simulink model "audio"  (Simulink 6.6)
settings: Solver=VariableStepDiscrete  StartTime=0.0  StopTime=15  RelTol=1e-3
PreLoadFcn:
  | Tsysclk=1/24000000;
  | Fs = 48000;
  | code_a = [0 0 0 0 1];
  | code_b = [0 0 0 1 0];
  | code_c = [0 0 0 1 1];
  | code_d = [1 0 1 1 1];
  | sum_filter_taps = ones(1,31);
libraries: xbsIndex_r4 x57, dspwin32 x2, simulink x1
settings Model: Creator=lcrockett  LastModifiedBy=lcrockett
settings OptimizationCC: InlineParams=on  InlineInvariantSignals=on
settings DebuggingCC: SignalResolutionControl=TryResolveAllWithWarning  MultiTaskDSMMsg=warning  MultiTaskCondExecSysMsg=none  StrictBusMsg=None
settings HardwareCC: TargetHWDeviceType=32-bit Generic  ProdEqTarget=off
settings RTWCC: IncludeERTFirstTime=on

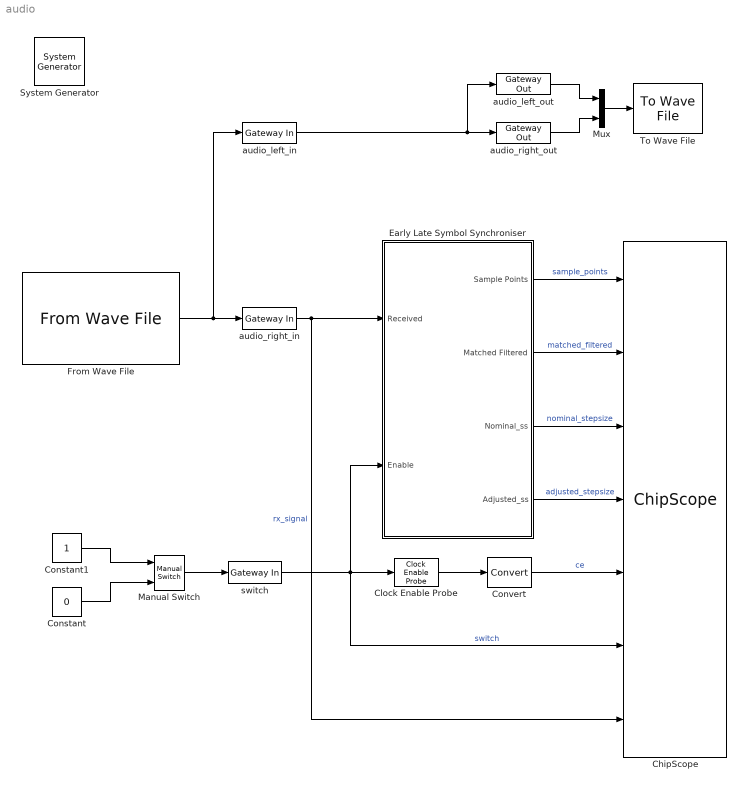
== system audio ==
  " System Generator" : xbsIndex_r4/ System Generator  Tag=genX  SystemSampleTime=-1  xilinxfamily=virtex2p  part=xc2vp30  speed=-7  package=ff896  synthesis_tool=XST  clock_wrapper=Clock Enables  directory=./audio_earlylate  testbench=off  simulink_period=Tsysclk  sysclk_period=50  dcm_input_clock_period=100  incr_netlist=off  trim_vbits=Everywhere in SubSystem  dbl_ovrd=According to Block Masks  core_generation=According to Block Masks  run_coregen=off  deprecated_control=off  eval_field=0  block_type=sysgen
      settings: block_version=8.2
  ChipScope : xbsIndex_r4/ChipScope  num_trig_ports=7  current_port=5  show_trig_port=0  match_units=1  match_type=Extended  data_is_trigger=on  num_data_ports=4  data_depth=16384  SRL16s=on  match_type_t0=1  match_type_t1=3  match_type_t2=3  match_type_t3=3  match_type_t4=3  match_type_t5=3  match_type_t6=3  match_type_t7=1  match_type_t8=1  match_type_t9=1  match_type_t10=1  match_type_t11=1  match_type_t12=1  match_type_t13=1  match_type_t14=1  match_type_t15=1  match_units_t0=1  match_units_t1=1  match_units_t2=1  match_units_t3=1  match_units_t4=1  match_units_t5=1  match_units_t6=1  match_units_t7=1  match_units_t8=1  match_units_t9=1  match_units_t10=1  match_units_t11=1  match_units_t12=1  match_units_t13=1  match_units_t14=1  match_units_t15=1  dbl_ovrd=0  block_type=chipscope
      settings: infoedit="Enables run-time debugging and verification of signals by inserting ChipScope Pro ICON and ILA cores.<br><br>  Restrictions: <br>Only one ChipScope core can be instantiated in a System Generator design.This block cannot be used at the same time as JTAG hardware co-simulation.A design or subsystem containing a ChipScope block must have at least one output port."  block_version=10.1.2
  Clock Enable Probe : xbsIndex_r4/Clock Enable Probe  block_type=ceprobe
      settings: infoedit="Clock enable extractor.  Produces a Boolean output that mirrors the hardware clock enable associated with the input sample rate.<P><P>Hardware notes: in hardware this block costs nothing."  block_version=10.1.2
  Constant : Constant  Value=0  SampleTime=Tsysclk*500
  Constant1 : Constant  SampleTime=Tsysclk*500
  Convert : xbsIndex_r4/Convert  arith_type=Unsigned  n_bits=1  bin_pt=0  quantization=Truncate  overflow=Wrap  latency=0  dbl_ovrd=off  pipeline=off  block_type=convert
      settings: block_version=10.1.2
  Early Late Symbol Synchroniser : Subsystem
  From Wave File : dspwin32/From Wave File  FileName=baseband_audio  SamplesPerFrame=1  MinBufSize=128  dType=double  bLoop=off  timesToPlay=1  restartMode=immediately after last sample  firstSampleOutput=off  lastSampleOutput=off
  Manual Switch : simulink/Signal Routing/Manual Switch  SystemSampleTime=-1  sw=0  action=0  varsize=off
  Mux : Mux  Inputs=2
  To Wave File : dspwin32/To Wave File  filename=audio  sampleWidth=16  MinNumSamples=256
  audio_left_in : xbsIndex_r4/Gateway In  arith_type="Signed  (2's comp)"  n_bits=16  bin_pt=14  quantization="Round  (unbiased: +/- Inf)"  overflow=Saturate  period=Tsysclk*500  dbl_ovrd=off  timing_constraint=None  locs_specified=off  LOCs={}  block_type=gatewayin
      settings: infoedit="Gateway in block.  Converts inputs of type Simulink integer, double and fixed point to  Xilinx fixed point type.<P><P>Hardware notes:  In hardware these blocks become top level input ports."  xl_area=[0 0 0 0 16 0 0]  block_version=VER_STRING_GOES_HERE
  audio_left_out : xbsIndex_r4/Gateway Out  hdl_port=on  timing_constraint=None  locs_specified=off  LOCs={}  block_type=gatewayout
      settings: infoedit="Gateway out block.  Converts Xilinx fixed point inputs into ouputs of type Simulink integer, double, or fixed point.<P><P>Hardware notes:  In hardware these blocks become top level output ports or are discarded, depending on how they are configured."  xl_area=[0 0 0 0 16 0 0]  block_version=VER_STRING_GOES_HERE
  audio_right_in : xbsIndex_r4/Gateway In  arith_type="Signed  (2's comp)"  n_bits=16  bin_pt=14  quantization="Round  (unbiased: +/- Inf)"  overflow=Saturate  period=Tsysclk*500  dbl_ovrd=off  timing_constraint=None  locs_specified=off  LOCs={}  block_type=gatewayin
      settings: infoedit="Gateway in block.  Converts inputs of type Simulink integer, double and fixed point to  Xilinx fixed point type.<P><P>Hardware notes:  In hardware these blocks become top level input ports."  xl_area=[0 0 0 0 16 0 0]  block_version=VER_STRING_GOES_HERE
  audio_right_out : xbsIndex_r4/Gateway Out  hdl_port=on  timing_constraint=None  locs_specified=off  LOCs={}  block_type=gatewayout
      settings: infoedit="Gateway out block.  Converts Xilinx fixed point inputs into ouputs of type Simulink integer, double, or fixed point.<P><P>Hardware notes:  In hardware these blocks become top level output ports or are discarded, depending on how they are configured."  xl_area=[0 0 0 0 16 0 0]  block_version=VER_STRING_GOES_HERE
  switch : xbsIndex_r4/Gateway In  arith_type=Boolean  n_bits=16  bin_pt=14  quantization="Round  (unbiased: +/- Inf)"  overflow=Saturate  period=Tsysclk*500  dbl_ovrd=off  timing_constraint=None  locs_specified=off  LOCs={}  block_type=gatewayin
      settings: infoedit="Gateway in block.  Converts inputs of type Simulink integer, double and fixed point to  Xilinx fixed point type.<P><P>Hardware notes:  In hardware these blocks become top level input ports."  xl_area=[0 0 0 0 16 0 0]  block_version=VER_STRING_GOES_HERE
  wires:
  From Wave File/1 -> audio_left_in/1, audio_right_in/1
  audio_right_out/1 -> Mux/2
  audio_left_out/1 -> Mux/1
  Mux/1 -> To Wave File/1
  switch/1 -> Clock Enable Probe/1, Early Late Symbol Synchroniser/2(Enable), ChipScope/6  "switch"
  Manual Switch/1 -> switch/1
  Constant1/1 -> Manual Switch/1
  Constant/1 -> Manual Switch/2
  audio_left_in/1 -> audio_left_out/1, audio_right_out/1
  audio_right_in/1 -> Early Late Symbol Synchroniser/1(Received), ChipScope/7  "rx_signal"
  Clock Enable Probe/1 -> Convert/1
  Convert/1 -> ChipScope/5  "ce"
  Early Late Symbol Synchroniser/1(Sample Points) -> ChipScope/1  "sample_points"
  Early Late Symbol Synchroniser/2(Matched Filtered) -> ChipScope/2  "matched_filtered"
  Early Late Symbol Synchroniser/3(Nominal_ss) -> ChipScope/3  "nominal_stepsize"
  Early Late Symbol Synchroniser/4(Adjusted_ss) -> ChipScope/4  "adjusted_stepsize"

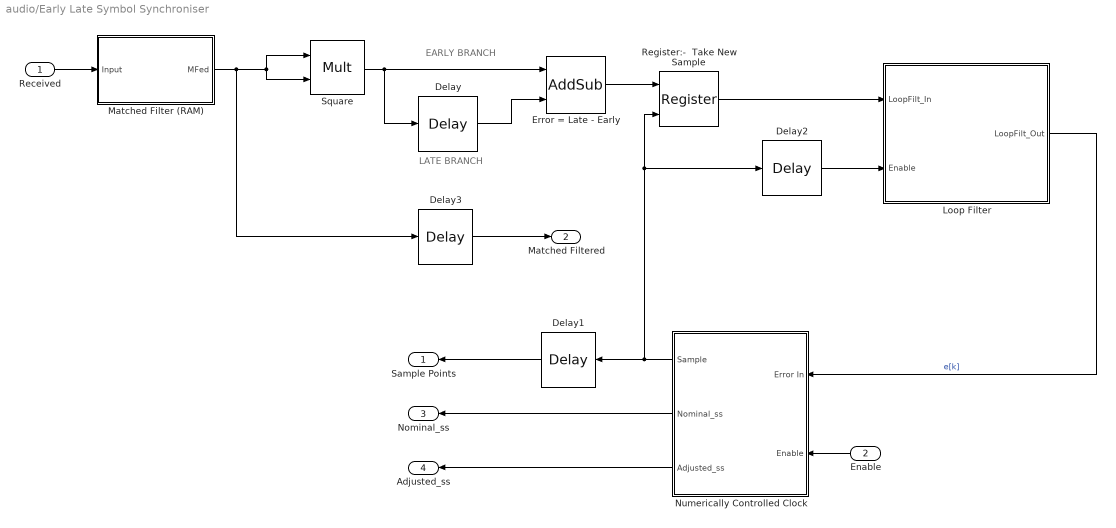
== system audio/Early Late Symbol Synchroniser ==
  note: LATE BRANCH
  note: EARLY BRANCH
  Received : Inport
  Enable : Inport  Orientation=left  Port=2
  Delay : xbsIndex_r4/Delay  en=off  latency=10  dbl_ovrd=off  reg_retiming=off  block_type=delay
      settings: block_version=9.2.01
  Delay1 : xbsIndex_r4/Delay  Orientation=left  en=off  latency=10  dbl_ovrd=off  reg_retiming=off  block_type=delay
      settings: block_version=9.2.01
  Delay2 : xbsIndex_r4/Delay  en=off  latency=1  dbl_ovrd=off  reg_retiming=off  block_type=delay
      settings: block_version=9.2.01
  Delay3 : xbsIndex_r4/Delay  en=off  latency=5  dbl_ovrd=off  reg_retiming=off  block_type=delay
      settings: block_version=9.2.01
  Error = Late - Early : xbsIndex_r4/AddSub  mode=Subtraction  use_carryin=off  use_carryout=off  en=off  latency=0  precision=User Defined  arith_type="Signed  (2's comp)"  n_bits=16  bin_pt=14  quantization=Truncate  overflow=Wrap  dbl_ovrd=off  use_behavioral_HDL=off  pipelined=off  use_rpm=on  block_type=addsub
      settings: block_version=9.2.01
  Loop Filter : Subsystem  mask(Loop Filter Parameters){alpha_n=5, beta_n=9, phase_det_word=16, extend_wl=on}
      mask prompts: alpha_n "Alpha (bits to shift right by)"; beta_n "Beta (bits to shift right by)"; phase_det_word "Input wordlength"; extend_wl "Retain full precision?"
      mask help:
      | The loop filter contains two paths: a proportional path and an integral path. These are characterised by coefficients Alpha and Beta, respectively. Multiplications by these coefficients are both realised via shifts, for hardware efficiency reasons.
      |
      | Mask to be completed... not yet straight on the wordlength implications and the choices that should be presented via the mask.
      mask init:
      | if extend_wl == true
      |     alpha_shift_wl = phase_det_word + alpha_n;
      |     beta_shift_wl = phase_det_word + beta_n;
      | else
      |     alpha_shift_wl = phase_det_word;
      |     beta_shift_wl = phase_det_word;
      | end
  Matched Filter (RAM) : Subsystem  mask(Rectangular Matched Filter){N=20}
      mask prompts: N "Moving Average (N samples)"
      mask help: This acts as a moving average filter of length N samples.
  Numerically Controlled Clock : Subsystem  Orientation=left  mask(Numerically Controlled Clock (NCC)){N=256, F_res=0.0001, F_nom=Fs/20, F_s=Fs}
      mask prompts: N "Counter Size"; F_res "Desired Frequency Resolution (Hz)"; F_nom "Nominal Rate/Frequency"; F_s "Sampling Frequency (Hz)"
      mask help: This component operates similarly to an NCO. Its "centre" rate is supplied by the user, defining the nominal step size applied to an accumulator. In operation, the control input "Error In" supplies a step size adjustment, which is applied to the nominal step size and input to an accumulator. When the accumulator wraps, a sample is taken (i.e. a single cycle 1 output).
      mask init:
      | delta_mu_des = (F_res * N) / F_s;
      | fract_bits = ceil(abs((log10(delta_mu_des) / log10(2))));
      | whole_bits = round(log(N)/log(2));
      | mu_nom = (F_nom * N) / F_s;
      | F_res_act = F_s / ((2^fract_bits) * N);
  Register:-  Take New Sample : xbsIndex_r4/Register  init=0  rst=off  en=on  dbl_ovrd=off  block_type=register
      settings: block_version=9.2.01
  Square : xbsIndex_r4/Mult  precision=User Defined  arith_type="Signed  (2's comp)"  n_bits=16  bin_pt=14  quantization=Truncate  overflow=Wrap  en=off  latency=0  dbl_ovrd=off  use_behavioral_HDL=off  use_embedded=on  opt=Speed  optimum_pipeline=off  pipeline=on  use_rpm=on  placement_style=Triangular  block_type=mult
      settings: infoedit=Hardware notes: To use the internal pipeline stage of the dedicated multiplier you must select 'Pipeline for maximum performance'.  block_version=9.2.01
  Sample Points : Outport  Orientation=left
  Matched Filtered : Outport  Port=2
  Nominal_ss : Outport  Orientation=left  Port=3
  Adjusted_ss : Outport  Orientation=left  Port=4
  wires:
  Loop Filter/1(LoopFilt_Out) -> Numerically Controlled Clock/1(Error In)  "e[k]"
  Register:-  Take New Sample/1 -> Loop Filter/1(LoopFilt_In)
  Delay/1 -> Error = Late - Early/2
  Error = Late - Early/1 -> Register:-  Take New Sample/1
  Matched Filter (RAM)/1(MFed) -> Square/1, Square/2, Delay3/1
  Square/1 -> Error = Late - Early/1, Delay/1
  Numerically Controlled Clock/1(Sample) -> Delay1/1, Register:-  Take New Sample/2, Delay2/1
  Delay2/1 -> Loop Filter/2(Enable)
  Received/1 -> Matched Filter (RAM)/1(Input)
  Enable/1 -> Numerically Controlled Clock/2(Enable)
  Delay1/1 -> Sample Points/1
  Numerically Controlled Clock/2(Nominal_ss) -> Nominal_ss/1
  Numerically Controlled Clock/3(Adjusted_ss) -> Adjusted_ss/1
  Delay3/1 -> Matched Filtered/1

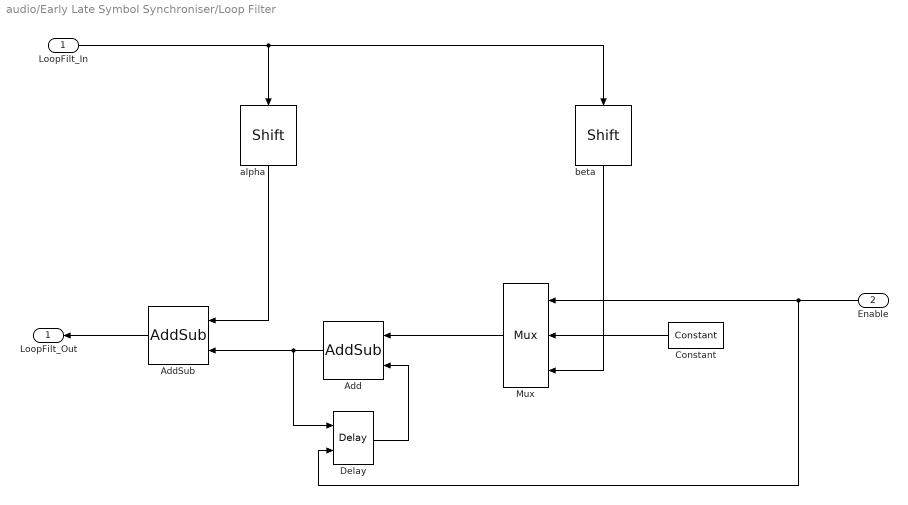
== system audio/Early Late Symbol Synchroniser/Loop Filter ==
  LoopFilt_In : Inport
  Enable : Inport  Orientation=left  Port=2
  Add : xbsIndex_r4/AddSub  Orientation=left  mode=Addition  use_carryin=off  use_carryout=off  en=off  latency=0  precision=User Defined  arith_type="Signed  (2's comp)"  n_bits=40  bin_pt=20  quantization="Round  (unbiased: +/- Inf)"  overflow=Wrap  dbl_ovrd=off  use_behavioral_HDL=off  pipelined=off  use_rpm=on  block_type=addsub
      settings: block_version=9.2.01
  AddSub : xbsIndex_r4/AddSub  Orientation=left  mode=Addition  use_carryin=off  use_carryout=off  en=off  latency=0  precision=Full  arith_type="Signed  (2's comp)"  n_bits=20  bin_pt=14  quantization="Round  (unbiased: +/- Inf)"  overflow=Wrap  dbl_ovrd=off  use_behavioral_HDL=off  pipelined=off  use_rpm=on  block_type=addsub
      settings: block_version=9.2.01
  Constant : xbsIndex_r4/Constant  Orientation=left  arith_type=Signed (2's comp)  const=0  n_bits=2  bin_pt=0  explicit_period=off  period=1  equ=P=C  opselect=C  inp2=PCIN>>17  opr=+  inp1=P  carry=CIN  dbl_ovrd=off  block_type=constant
      settings: block_version=9.2.01
  Delay : xbsIndex_r4/Delay  en=on  latency=1  dbl_ovrd=off  reg_retiming=off  block_type=delay
      settings: block_version=9.2.01
  Mux : xbsIndex_r4/Mux  Orientation=left  inputs=2  en=off  latency=0  precision=Full  arith_type=Unsigned  n_bits=16  bin_pt=14  quantization=Truncate  overflow=Wrap  dbl_ovrd=off  block_type=mux
      settings: block_version=9.2.01
  alpha : xbsIndex_r4/Shift  Orientation=down  shift_dir=Right  shift_bits=alpha_n  en=off  latency=0  precision=User Defined  arith_type="Signed  (2's comp)"  n_bits=alpha_shift_wl  bin_pt=alpha_shift_wl-2  quantization="Round  (unbiased: +/- Inf)"  overflow=Wrap  dbl_ovrd=off  block_type=shift
      settings: block_version=9.2.01
  beta : xbsIndex_r4/Shift  Orientation=down  shift_dir=Right  shift_bits=beta_n  en=off  latency=0  precision=User Defined  arith_type="Signed  (2's comp)"  n_bits=beta_shift_wl  bin_pt=beta_shift_wl-2  quantization="Round  (unbiased: +/- Inf)"  overflow=Wrap  dbl_ovrd=off  block_type=shift
      settings: block_version=9.2.01
  LoopFilt_Out : Outport  Orientation=left
  wires:
  Add/1 -> AddSub/2, Delay/1
  alpha/1 -> AddSub/1
  Delay/1 -> Add/2
  LoopFilt_In/1 -> alpha/1, beta/1
  AddSub/1 -> LoopFilt_Out/1
  beta/1 -> Mux/3
  Mux/1 -> Add/1
  Enable/1 -> Mux/1, Delay/2
  Constant/1 -> Mux/2

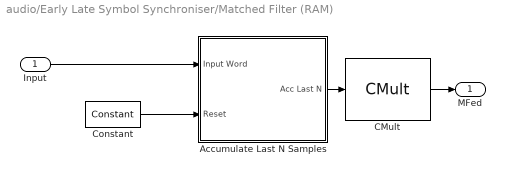
== system audio/Early Late Symbol Synchroniser/Matched Filter (RAM) ==
  Input : Inport
  Accumulate Last N Samples : Subsystem  mask(Sliding Accumulator){N=N, Wbits=16, Bpoint=14}
      mask prompts: N "Accumulate window (samples)"; Wbits "Input wordlength"; Bpoint "Binary point"
      mask help:
      | This block accumulates over a specified number of samples.
      |
      | Internal and output wordlengths are defined by the wordlength of the input, and the accumulator window.
  CMult : xbsIndex_r4/CMult  const=1/N  const_n_bits=16  const_bin_pt=14  en=off  latency=0  precision=User Defined  arith_type="Signed  (2's comp)"  n_bits=16  bin_pt=14  quantization=Truncate  overflow=Wrap  dbl_ovrd=off  use_behavioral_HDL=off  mem_type=Distributed RAM  placement_style=Rectangular Shape  pipeline=off  use_rpm=off  block_type=cmult
      settings: block_version=10.1
  Constant : xbsIndex_r4/Constant  arith_type=Boolean  const=0  n_bits=16  bin_pt=14  explicit_period=on  period=1/Fs  equ=P=C  opselect=C  inp2=PCIN>>17  opr=+  inp1=P  carry=CIN  dbl_ovrd=off  block_type=constant
      settings: block_version=10.1.2
  MFed : Outport
  wires:
  Accumulate Last N Samples/1(Acc Last N) -> CMult/1
  Input/1 -> Accumulate Last N Samples/1(Input Word)
  CMult/1 -> MFed/1
  Constant/1 -> Accumulate Last N Samples/2(Reset)

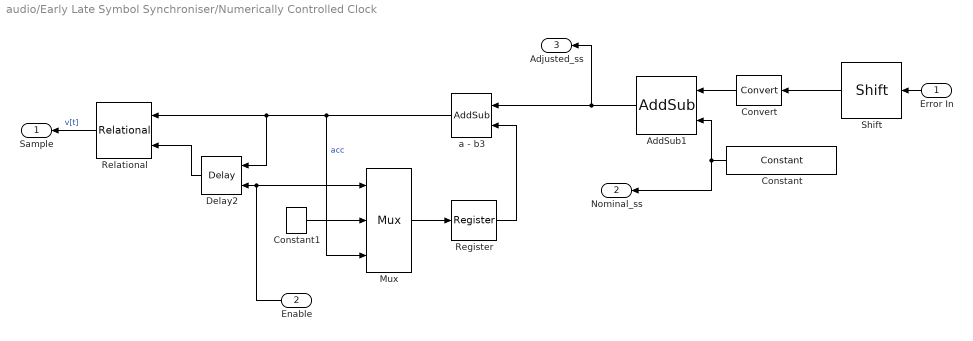
== system audio/Early Late Symbol Synchroniser/Numerically Controlled Clock ==
  Error In : Inport  Orientation=left
  Enable : Inport  Orientation=left  Port=2
  AddSub1 : xbsIndex_r4/AddSub  Orientation=left  mode=Addition  use_carryin=off  use_carryout=off  en=off  latency=0  precision=User Defined  arith_type=Unsigned  n_bits=whole_bits + fract_bits  bin_pt=fract_bits  quantization="Round  (unbiased: +/- Inf)"  overflow=Wrap  dbl_ovrd=off  use_behavioral_HDL=off  pipelined=off  use_rpm=on  block_type=addsub
      settings: block_version=9.2.01
  Constant : xbsIndex_r4/Constant  Orientation=left  arith_type=Unsigned  const=mu_nom  n_bits=whole_bits + fract_bits  bin_pt=fract_bits  explicit_period=on  period=1/Fs  equ=P=C  opselect=C  inp2=PCIN>>17  opr=+  inp1=P  carry=CIN  dbl_ovrd=off  block_type=constant
      settings: block_version=9.2.01
  Constant1 : xbsIndex_r4/Constant  arith_type=Signed (2's comp)  const=0  n_bits=16  bin_pt=14  explicit_period=on  period=1/Fs  equ=P=C  opselect=C  inp2=PCIN>>17  opr=+  inp1=P  carry=CIN  dbl_ovrd=off  block_type=constant
      settings: block_version=10.1.2
  Convert : xbsIndex_r4/Convert  Orientation=left  arith_type="Signed  (2's comp)"  n_bits=whole_bits+fract_bits  bin_pt=fract_bits  quantization=Truncate  overflow=Wrap  latency=0  dbl_ovrd=off  pipeline=off  block_type=convert
      settings: block_version=9.2.01
  Delay2 : xbsIndex_r4/Delay  Orientation=left  en=on  latency=1  dbl_ovrd=off  reg_retiming=off  block_type=delay
      settings: block_version=9.2.01
  Mux : xbsIndex_r4/Mux  inputs=2  en=off  latency=0  precision=Full  arith_type=Unsigned  n_bits=16  bin_pt=14  quantization=Truncate  overflow=Wrap  dbl_ovrd=off  block_type=mux
      settings: block_version=10.1.2
  Register : xbsIndex_r4/Register  init=0  rst=off  en=off  dbl_ovrd=off  block_type=register
      settings: block_version=10.1.2
  Relational : xbsIndex_r4/Relational  Orientation=left  mode=a<b  en=off  latency=1  dbl_ovrd=off  block_type=relational
      settings: block_version=9.2.01
  Shift : xbsIndex_r4/Shift  Orientation=left  shift_dir=Left  shift_bits=4  en=off  latency=0  precision=Full  arith_type="Signed  (2's comp)"  n_bits=16  bin_pt=14  quantization=Truncate  overflow=Wrap  dbl_ovrd=off  block_type=shift
      settings: block_version=9.2.01
  a - b3 : xbsIndex_r4/AddSub  Orientation=left  mode=Addition  use_carryin=off  use_carryout=off  en=off  latency=0  precision=User Defined  arith_type=Unsigned  n_bits=whole_bits + fract_bits  bin_pt=fract_bits  quantization=Truncate  overflow=Wrap  dbl_ovrd=off  use_behavioral_HDL=off  pipelined=off  use_rpm=on  block_type=addsub
      settings: block_version=9.2.01
  Sample : Outport  Orientation=left
  Nominal_ss : Outport  Orientation=left  Port=2
  Adjusted_ss : Outport  Orientation=left  Port=3
  wires:
  a - b3/1 -> Delay2/1, Relational/1, Mux/3  "acc"
  Register/1 -> a - b3/2
  AddSub1/1 -> a - b3/1, Adjusted_ss/1
  Constant/1 -> AddSub1/2, Nominal_ss/1
  Delay2/1 -> Relational/2
  Error In/1 -> Shift/1
  Relational/1 -> Sample/1  "v[t]"
  Enable/1 -> Mux/1, Delay2/2
  Convert/1 -> AddSub1/1
  Shift/1 -> Convert/1
  Mux/1 -> Register/1
  Constant1/1 -> Mux/2

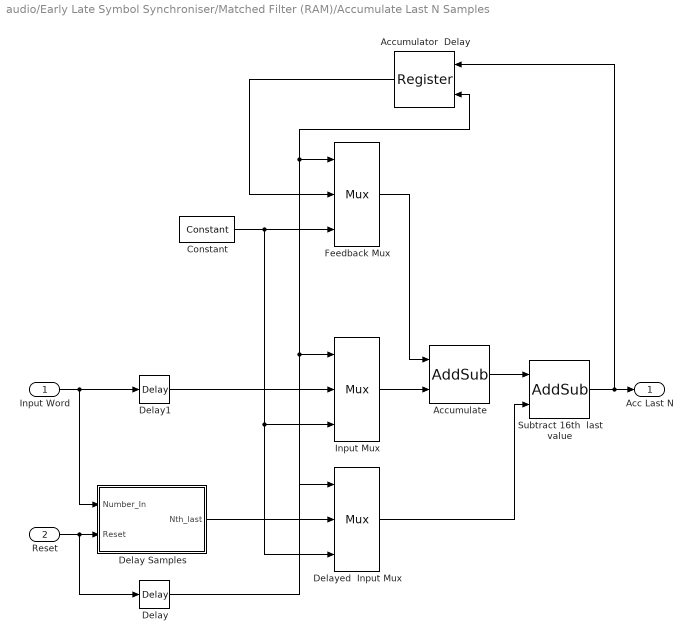
== system audio/Early Late Symbol Synchroniser/Matched Filter (RAM)/Accumulate Last N Samples ==
  Input Word : Inport
  Reset : Inport  Port=2
  Accumulate : xbsIndex_r4/AddSub  mode=Addition  use_carryin=off  use_carryout=off  en=off  latency=0  precision=User Defined  arith_type="Signed  (2's comp)"  n_bits=Wbits+ceil(log2(N))  bin_pt=Bpoint  quantization=Truncate  overflow=Wrap  dbl_ovrd=off  use_behavioral_HDL=off  pipelined=off  use_rpm=on  block_type=addsub
      settings: xl_area=[9 0 0 16 0 0 0]  block_version=9.2.01
  Accumulator  Delay : xbsIndex_r4/Register  Orientation=left  init=0  rst=on  en=off  dbl_ovrd=off  block_type=register
      settings: xl_area=[8 16 0 0 0 0 0]  block_version=9.2.01
  Constant : xbsIndex_r4/Constant  arith_type=Signed (2's comp)  const=0  n_bits=2  bin_pt=0  explicit_period=off  period=1  equ=P=C  opselect=C  inp2=PCIN>>17  opr=+  inp1=P  carry=CIN  dbl_ovrd=off  block_type=constant
      settings: block_version=9.2.01
  Delay : xbsIndex_r4/Delay  en=off  latency=1  dbl_ovrd=off  reg_retiming=off  block_type=delay
      settings: block_version=9.2.01
  Delay Samples : Subsystem  mask(Parameterisable Delay){D=N}
      mask prompts: D "Samples delay"
      mask help: A dual-port RAM is used to synthesise a resettable delay line of the specified number of samples.
  Delay1 : xbsIndex_r4/Delay  en=off  latency=1  dbl_ovrd=off  reg_retiming=off  block_type=delay
      settings: block_version=9.2.01
  Delayed  Input Mux : xbsIndex_r4/Mux  inputs=2  en=off  latency=0  precision=Full  arith_type=Unsigned  n_bits=16  bin_pt=14  quantization=Truncate  overflow=Wrap  dbl_ovrd=off  block_type=mux
      settings: xl_area=[8 0 0 16 0 0 0]  block_version=9.2.01
  Feedback Mux : xbsIndex_r4/Mux  inputs=2  en=off  latency=0  precision=Full  arith_type=Unsigned  n_bits=16  bin_pt=14  quantization=Truncate  overflow=Wrap  dbl_ovrd=off  block_type=mux
      settings: xl_area=[8 0 0 16 0 0 0]  block_version=9.2.01
  Input Mux : xbsIndex_r4/Mux  inputs=2  en=off  latency=0  precision=Full  arith_type=Unsigned  n_bits=16  bin_pt=14  quantization=Truncate  overflow=Wrap  dbl_ovrd=off  block_type=mux
      settings: xl_area=[8 0 0 16 0 0 0]  block_version=9.2.01
  Subtract 16th  last value : xbsIndex_r4/AddSub  mode=Subtraction  use_carryin=off  use_carryout=off  en=off  latency=0  precision=User Defined  arith_type="Signed  (2's comp)"  n_bits=Wbits+ceil(log2(N))  bin_pt=Bpoint  quantization=Truncate  overflow=Wrap  dbl_ovrd=off  use_behavioral_HDL=off  pipelined=off  use_rpm=on  block_type=addsub
      settings: xl_area=[8 0 0 16 0 0 0]  block_version=9.2.01
  Acc Last N : Outport
  wires:
  Input Word/1 -> Delay1/1, Delay Samples/1(Number_In)
  Accumulate/1 -> Subtract 16th  last value/1
  Reset/1 -> Delay/1, Delay Samples/2(Reset)
  Subtract 16th  last value/1 -> Accumulator  Delay/1, Acc Last N/1
  Accumulator  Delay/1 -> Feedback Mux/2
  Feedback Mux/1 -> Accumulate/1
  Constant/1 -> Feedback Mux/3, Input Mux/3, Delayed  Input Mux/3
  Input Mux/1 -> Accumulate/2
  Delayed  Input Mux/1 -> Subtract 16th  last value/2
  Delay Samples/1(Nth_last) -> Delayed  Input Mux/2
  Delay/1 -> Input Mux/1, Delayed  Input Mux/1, Feedback Mux/1, Accumulator  Delay/2
  Delay1/1 -> Input Mux/2

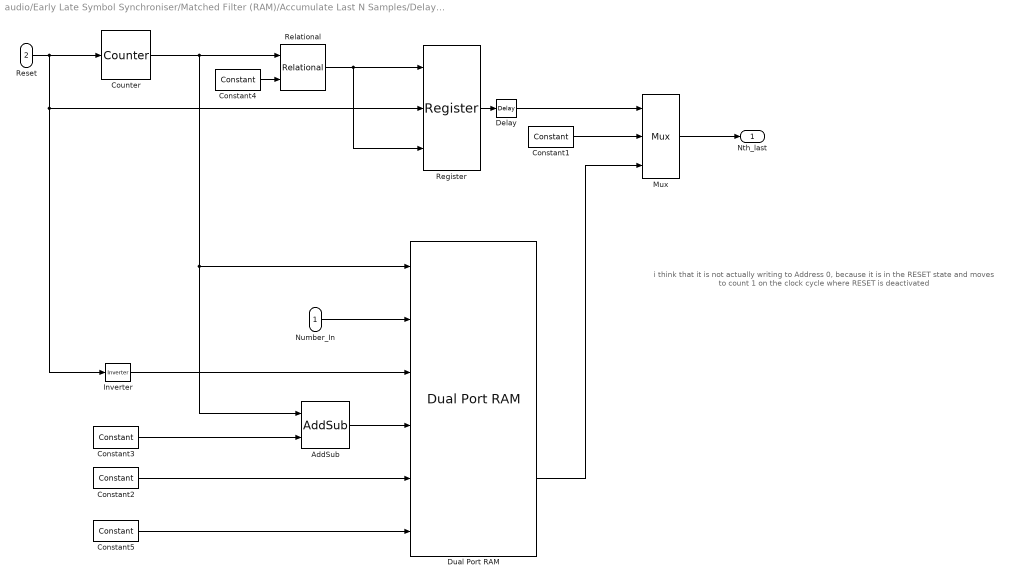
== system audio/Early Late Symbol Synchroniser/Matched Filter (RAM)/Accumulate Last N Samples/Delay Samples ==
  note: i think that it is not actually writing to Address 0, because it is in
      | the RESET state and moves to count 1 on the clock cycle where RESET is deactivated
  Number_In : Inport
  Reset : Inport  Port=2
  AddSub : xbsIndex_r4/AddSub  mode=Subtraction  use_carryin=off  use_carryout=off  en=off  latency=0  precision=User Defined  arith_type=Unsigned  n_bits=ceil(log2(D)+1)  bin_pt=0  quantization=Truncate  overflow=Wrap  dbl_ovrd=off  use_behavioral_HDL=off  pipelined=off  use_rpm=on  block_type=addsub
      settings: block_version=9.2.01
  Constant1 : xbsIndex_r4/Constant  arith_type=Signed (2's comp)  const=0  n_bits=2  bin_pt=0  explicit_period=off  period=1  equ=P=C  opselect=C  inp2=PCIN>>17  opr=+  inp1=P  carry=CIN  dbl_ovrd=off  block_type=constant
      settings: block_version=9.2.01
  Constant2 : xbsIndex_r4/Constant  arith_type=Signed (2's comp)  const=0  n_bits=16  bin_pt=14  explicit_period=off  period=1  equ=P=C  opselect=C  inp2=PCIN>>17  opr=+  inp1=P  carry=CIN  dbl_ovrd=off  block_type=constant
      settings: block_version=9.2.01
  Constant3 : xbsIndex_r4/Constant  arith_type=Unsigned  const=D  n_bits=ceil(log2(D)+1)  bin_pt=0  explicit_period=off  period=1  equ=P=C  opselect=C  inp2=PCIN>>17  opr=+  inp1=P  carry=CIN  dbl_ovrd=off  block_type=constant
      settings: block_version=9.2.01
  Constant4 : xbsIndex_r4/Constant  arith_type=Unsigned  const=D-1  n_bits=ceil(log2(D))  bin_pt=0  explicit_period=off  period=1  equ=P=C  opselect=C  inp2=PCIN>>17  opr=+  inp1=P  carry=CIN  dbl_ovrd=off  block_type=constant
      settings: block_version=9.2.01
  Constant5 : xbsIndex_r4/Constant  arith_type=Boolean  const=0  n_bits=ceil(log2(D)+1)  bin_pt=0  explicit_period=off  period=1  equ=P=C  opselect=C  inp2=PCIN>>17  opr=+  inp1=P  carry=CIN  dbl_ovrd=off  block_type=constant
      settings: block_version=9.2.01
  Counter : xbsIndex_r4/Counter  cnt_type=Free Running  cnt_to=Inf  operation=Up  start_count=0  cnt_by_val=1  arith_type=Unsigned  n_bits=ceil(log2(D)+1)  bin_pt=0  load_pin=off  rst=on  en=off  explicit_period=on  period=1/Fs  dbl_ovrd=off  use_behavioral_HDL=off  use_rpm=off  block_type=counter
      settings: block_version=9.2.01
  Delay : xbsIndex_r4/Delay  en=off  latency=1  dbl_ovrd=off  reg_retiming=off  block_type=delay
      settings: block_version=9.2.01
  Dual Port RAM : xbsIndex_r4/Dual Port RAM  depth=2^ceil(log2(D)+1)  initVector=zeros(1,ceil(log2(D)+1))  distributed_mem=Block RAM  init_a=0  init_b=0  rst_a=off  rst_b=off  en_a=off  en_b=off  latency=1  write_mode_A=Read After Write  write_mode_B=Read After Write  dbl_ovrd=off  optimize=Area  use_rpm=on  block_type=dpram
      settings: block_version=9.2.01
  Inverter : xbsIndex_r4/Inverter  en=off  latency=0  dbl_ovrd=off  block_type=inv
      settings: block_version=9.2.01
  Mux : xbsIndex_r4/Mux  inputs=2  en=off  latency=0  precision=Full  arith_type=Unsigned  n_bits=16  bin_pt=14  quantization=Truncate  overflow=Wrap  dbl_ovrd=off  block_type=mux
      settings: block_version=9.2.01
  Register : xbsIndex_r4/Register  init=0  rst=on  en=on  dbl_ovrd=off  block_type=register
      settings: block_version=9.2.01
  Relational : xbsIndex_r4/Relational  mode=a=b  en=off  latency=0  dbl_ovrd=off  block_type=relational
      settings: block_version=9.2.01
  Nth_last : Outport
  wires:
  Reset/1 -> Inverter/1, Register/2, Counter/1
  Number_In/1 -> Dual Port RAM/2
  Counter/1 -> AddSub/1, Dual Port RAM/1, Relational/1
  Relational/1 -> Register/1, Register/3
  Register/1 -> Delay/1
  Dual Port RAM/2 -> Mux/3
  Constant1/1 -> Mux/2
  Mux/1 -> Nth_last/1
  Constant4/1 -> Relational/2
  AddSub/1 -> Dual Port RAM/4
  Constant3/1 -> AddSub/2
  Inverter/1 -> Dual Port RAM/3
  Delay/1 -> Mux/1
  Constant2/1 -> Dual Port RAM/5
  Constant5/1 -> Dual Port RAM/6
